simulink model "inerter_NL2"  (R2024b)
settings: Solver=ode1be  StartTime=0.0  StopTime=20  FixedStep=0.001  MaxStep=1e-2  MinStep=1e-12  RelTol=1e-6  AbsTol=1e-6
libraries: fl_lib x19, nesl_utility x7, simulink x1
settings Model: Creator=yl14470  LastModifiedBy=vzlat
settings SolverCC: MaxConsecutiveZCs=10000  ZeroCrossAlgorithm=Adaptive
settings DebuggingCC: IgnoredZcDiagnostic=none
settings RTWCC: GPUComputeCapability=3.5

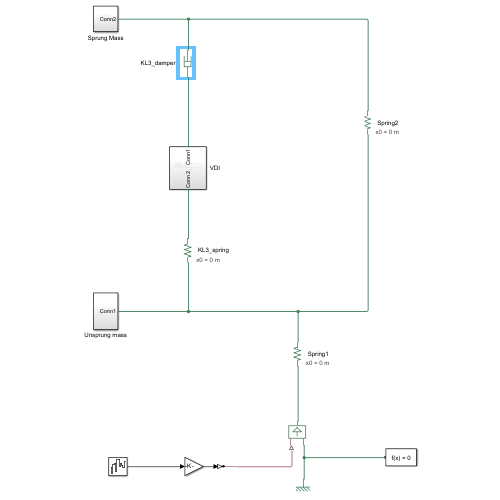
[thumbnail: Simulink's stored preview of the top-level diagram]
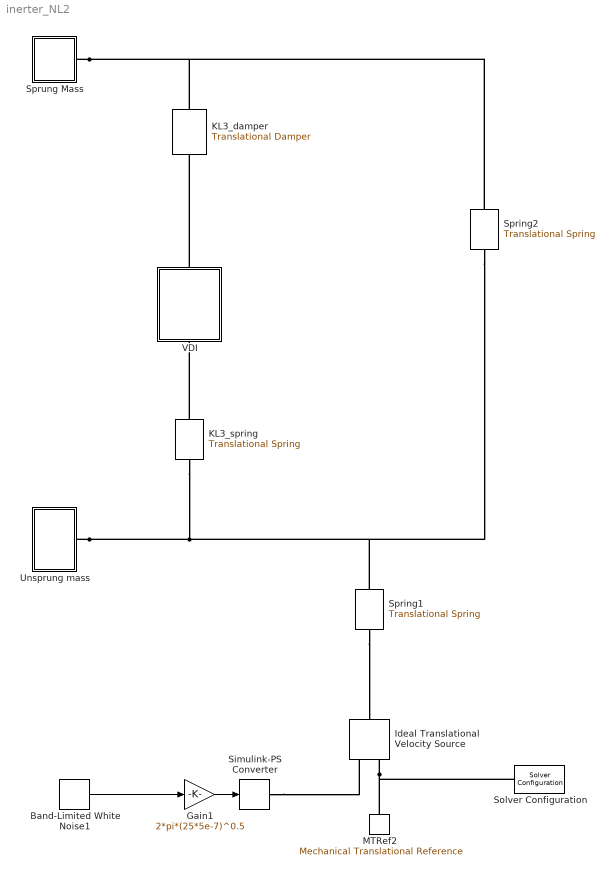
== system inerter_NL2 ==
  Band-Limited White Noise1 : simulink/Sources/Band-Limited White Noise  Cov=1  Ts=0.01  seed=[23341]
  Gain1 : Gain  Gain=2*pi*(25*5e-7)^0.5
  Ideal Translational Velocity Source : fl_lib/Mechanical/Mechanical Sources/Ideal Translational Velocity Source
  KL3_damper : fl_lib/Mechanical/Translational Elements/Translational Damper  D=962 N*s/m  v_specify=off  v_priority=None  v=0 m/s  v_nominal_specify=off  v_nominal_value=1  v_nominal_unit=m/s  f_specify=off  f_priority=None  f=0 N  f_nominal_specify=off  f_nominal_value=1  f_nominal_unit=N
  KL3_spring : fl_lib/Mechanical/Translational Elements/Translational Spring  spr_rate=10808 N/m  v_specify=off  v_priority=High  v=0 m/s  v_nominal_specify=off  v_nominal_value=1  v_nominal_unit=m/s  f_specify=off  f_priority=High  f=0 N  f_nominal_specify=off  f_nominal_value=1  f_nominal_unit=N  x_specify=on  x_priority=High  x=0 m  x_nominal_specify=off  x_nominal_value=1  x_nominal_unit=m
      settings: AttributesFormatString=x0 = %<x> %<x_unit>
  MTRef2 : fl_lib/Mechanical/Translational Elements/Mechanical Translational Reference
  Simulink-PS Converter : nesl_utility/Simulink-PS Converter  PhysicalDomain=network_engine_domain  SubClassName=ps_input  LeftPortType=input  RightPortType=output  PseudoPeriodic=off  Frequencies=[]  NoiseDistribution=none  NoiseParameters=[]  Unit=m/s  AffineConversion=off  FilteringAndDerivatives=filter  SimscapeFilterOrder=1  InputFilterTimeConstant=0.001  UdotUserProvided=0
  Solver Configuration : nesl_utility/Solver Configuration  PhysicalDomain=network_engine_domain  SubClassName=solver  LeftPortType=input  RightPortType=generic  Tones=[]  Harmonics=[]  SimulateNoise=off  Profile=off  UseLocalSampling=off  EnableSwitchedLinearOptims=on  FrequencyDomain=off  UseCCode=off  RelTol=0.001  AbsTol=1e-06  MinStep=1e-09  ToWorkspace=off  RevertToSquareIcSolve=off  NumHomotopyIterations=100  PhasorMode=off  PhasorModeNumHarmonics=1  ConsistencySolver=NEWTON_FTOL  IndexReductionMethod=DerivativeReplacement  DoDC=off  ResidualTolerance=1e-9  ConsistencyTolSource=GLOBAL  ConsistencyAbsTol=0.001  ConsistencyRelTol=0.001  ConsistencyTolFactor=0.001  UseLocalSolver=off  LocalSolverChoice=NE_BACKWARD_EULER_ADVANCER  ResolveIndetEquations=on  FunctionEvalNumThread=1  LocalSolverSampleTime=.001  DoFixedCost=off  MaxNonlinIter=12  MaxModeIter=2  ComputeImpulses=off  ImpulseIterations=2  LinearAlgebra=Sparse  LinearAlgebraNumThread=0  EquationFormulation=NE_TIME_EF  DelaysMemoryBudget=1024  AutomaticFiltering=on  FilteringTimeConstant=0.001  PartitionStorageMethod=AS_NEEDED  PartitionMemoryBudget=1024  PartitionMethod=FAST  MultibodyUseLocalSolver=off  MultibodyLocalSolverChoice=ODE1  MultibodyLocalSolverSampleTime=0.001
  Spring1 : fl_lib/Mechanical/Translational Elements/Translational Spring  spr_rate=160000 N/m  v_specify=off  v_priority=High  v=0 m/s  v_nominal_specify=off  v_nominal_value=1  v_nominal_unit=m/s  f_specify=off  f_priority=High  f=0 N  f_nominal_specify=off  f_nominal_value=1  f_nominal_unit=N  x_specify=on  x_priority=High  x=0 m  x_nominal_specify=off  x_nominal_value=1  x_nominal_unit=m
      settings: AttributesFormatString=x0 = %<x> %<x_unit>
  Spring2 : fl_lib/Mechanical/Translational Elements/Translational Spring  spr_rate=16998.2107 N/m  v_specify=off  v_priority=High  v=0 m/s  v_nominal_specify=off  v_nominal_value=1  v_nominal_unit=m/s  f_specify=off  f_priority=High  f=0 N  f_nominal_specify=off  f_nominal_value=1  f_nominal_unit=N  x_specify=on  x_priority=High  x=0 m  x_nominal_specify=off  x_nominal_value=1  x_nominal_unit=m
      settings: AttributesFormatString=x0 = %<x> %<x_unit>
  Sprung Mass : Subsystem
  Unsprung mass : Subsystem
  VDI : Subsystem
  wires:
  Gain1/1 -> Simulink-PS Converter/1
  Band-Limited White Noise1/1 -> Gain1/1
  connections:
  Sprung Mass/RConn1 -- Spring2/LConn1 -- KL3_damper/LConn1
  Unsprung mass/RConn1 -- Spring1/LConn1 -- Spring2/RConn1 -- KL3_spring/RConn1
  Ideal Translational Velocity Source/RConn2 -- MTRef2/LConn1 -- Solver Configuration/RConn1
  Spring1/RConn1 -- Ideal Translational Velocity Source/LConn1
  Simulink-PS Converter/RConn1 -- Ideal Translational Velocity Source/RConn1
  KL3_spring/LConn1 -- VDI/LConn1
  VDI/RConn1 -- KL3_damper/RConn1

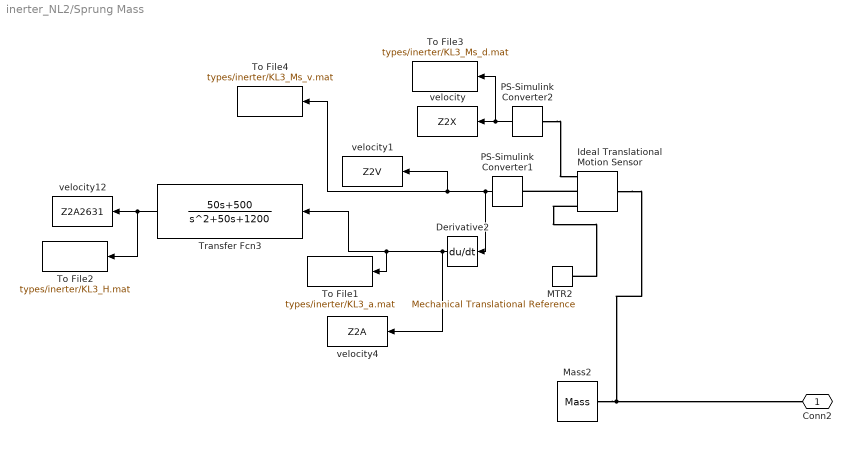
== system inerter_NL2/Sprung Mass ==
  Derivative2 : Derivative
  Ideal Translational Motion Sensor : fl_lib/Mechanical/Mechanical Sensors/Ideal Translational Motion Sensor  reference=foundation.enum.MeasurementReference.difference  acceleration_port=false  velocity_port=true  position_port=true  offset=0 m
  MTR2 : fl_lib/Mechanical/Translational Elements/Mechanical Translational Reference
  Mass2 : fl_lib/Mechanical/Translational Elements/Mass  mass=240 kg  num_ports=foundation.enum.numPorts2.one  v_specify=off  v_priority=High  v=0 m/s  v_nominal_specify=off  v_nominal_value=1  v_nominal_unit=m/s  f_specify=off  f_priority=High  f=0 N  f_nominal_specify=off  f_nominal_value=1  f_nominal_unit=N
  PS-Simulink Converter1 : nesl_utility/PS-Simulink Converter  PhysicalDomain=network_engine_domain  SubClassName=ps_output  LeftPortType=input  RightPortType=output  PseudoPeriodic=off  Frequencies=[]  VectorFormat=1-D array  Unit=1  AffineConversion=off
  PS-Simulink Converter2 : nesl_utility/PS-Simulink Converter  PhysicalDomain=network_engine_domain  SubClassName=ps_output  LeftPortType=input  RightPortType=output  PseudoPeriodic=off  Frequencies=[]  VectorFormat=1-D array  Unit=1  AffineConversion=off
  To File1 : ToFile  Filename=types/inerter/KL3_a.mat  MatrixName=Ms_acc  SaveFormat=Timeseries
  To File2 : ToFile  Filename=types/inerter/KL3_H.mat  MatrixName=H2631  SaveFormat=Timeseries
  To File3 : ToFile  Filename=types/inerter/KL3_Ms_d.mat  MatrixName=Ms_d  SaveFormat=Timeseries
  To File4 : ToFile  Filename=types/inerter/KL3_Ms_v.mat  MatrixName=Ms_v  SaveFormat=Timeseries
  Transfer Fcn3 : TransferFcn  Numerator=[0 50 500]  Denominator=[1 50 1200]
  velocity : ToWorkspace  VariableName=Z2X  SampleTime=-1
  velocity1 : ToWorkspace  VariableName=Z2V  SampleTime=-1
  velocity12 : ToWorkspace  VariableName=Z2A2631  SampleTime=-1
  velocity4 : ToWorkspace  VariableName=Z2A  SampleTime=-1
  Conn2 : PMIOPort  Side=Right
  wires:
  Transfer Fcn3/1 -> To File2/1, velocity12/1
  PS-Simulink Converter1/1 -> Derivative2/1, To File4/1, velocity1/1
  Derivative2/1 -> To File1/1, Transfer Fcn3/1, velocity4/1
  PS-Simulink Converter2/1 -> velocity/1, To File3/1
  connections:
  Ideal Translational Motion Sensor/RConn1 -- MTR2/LConn1
  Mass2/LConn1 -- Conn2/RConn1 -- Ideal Translational Motion Sensor/LConn1
  Ideal Translational Motion Sensor/RConn2 -- PS-Simulink Converter1/LConn1
  PS-Simulink Converter2/LConn1 -- Ideal Translational Motion Sensor/RConn3

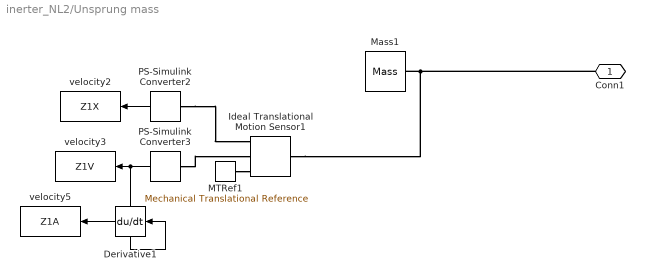
== system inerter_NL2/Unsprung mass ==
  Derivative1 : Derivative
  Ideal Translational Motion Sensor1 : fl_lib/Mechanical/Mechanical Sensors/Ideal Translational Motion Sensor  reference=foundation.enum.MeasurementReference.difference  acceleration_port=false  velocity_port=true  position_port=true  offset=0 m
  MTRef1 : fl_lib/Mechanical/Translational Elements/Mechanical Translational Reference
  Mass1 : fl_lib/Mechanical/Translational Elements/Mass  mass=36 kg  num_ports=foundation.enum.numPorts2.one  v_specify=off  v_priority=High  v=0 m/s  v_nominal_specify=off  v_nominal_value=1  v_nominal_unit=m/s  f_specify=off  f_priority=High  f=0 N  f_nominal_specify=off  f_nominal_value=1  f_nominal_unit=N
  PS-Simulink Converter2 : nesl_utility/PS-Simulink Converter  PhysicalDomain=network_engine_domain  SubClassName=ps_output  LeftPortType=input  RightPortType=output  PseudoPeriodic=off  Frequencies=[]  VectorFormat=1-D array  Unit=1  AffineConversion=off
  PS-Simulink Converter3 : nesl_utility/PS-Simulink Converter  PhysicalDomain=network_engine_domain  SubClassName=ps_output  LeftPortType=input  RightPortType=output  PseudoPeriodic=off  Frequencies=[]  VectorFormat=1-D array  Unit=1  AffineConversion=off
  velocity2 : ToWorkspace  VariableName=Z1X  SampleTime=-1
  velocity3 : ToWorkspace  VariableName=Z1V  SampleTime=-1
  velocity5 : ToWorkspace  VariableName=Z1A  SampleTime=-1
  Conn1 : PMIOPort  Side=Right
  wires:
  PS-Simulink Converter3/1 -> velocity3/1, Derivative1/1
  Derivative1/1 -> velocity5/1
  PS-Simulink Converter2/1 -> velocity2/1
  connections:
  Mass1/LConn1 -- Conn1/RConn1 -- Ideal Translational Motion Sensor1/LConn1
  MTRef1/LConn1 -- Ideal Translational Motion Sensor1/RConn1
  PS-Simulink Converter3/LConn1 -- Ideal Translational Motion Sensor1/RConn2
  PS-Simulink Converter2/LConn1 -- Ideal Translational Motion Sensor1/RConn3

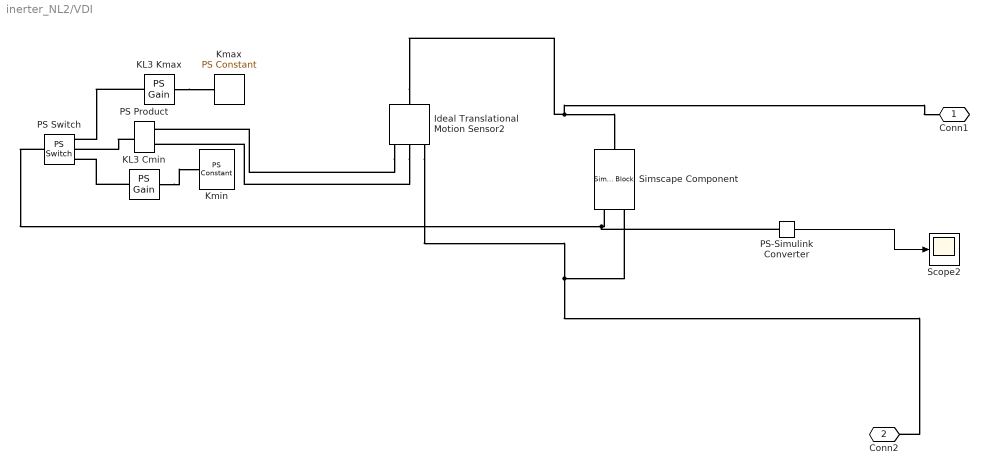
== system inerter_NL2/VDI ==
  Ideal Translational Motion Sensor2 : fl_lib/Mechanical/Mechanical Sensors/Ideal Translational Motion Sensor  reference=foundation.enum.MeasurementReference.difference  acceleration_port=false  velocity_port=true  position_port=true  offset=0 m
  KL3 Cmin : fl_lib/Physical Signals/Functions/PS Gain  gain=1
  KL3 Kmax : fl_lib/Physical Signals/Functions/PS Gain  gain=1
  Kmax : fl_lib/Physical Signals/Sources/PS Constant  constant=177 kg
  Kmin : fl_lib/Physical Signals/Sources/PS Constant  constant=68 kg
  PS Product : fl_lib/Physical Signals/Functions/PS Product
  PS Switch : fl_lib/Physical Signals/Nonlinear Operators/PS Switch  Threshold=0 m^2/s
      settings: InternalSimscapePortConfiguration="{\"Bottom\":[],\"Left\":[{\"id\":\"I1\",\"label\":\"\",\"type\":\"input\"},{\"id\":\"I2\",\"label\":\"\",\"type\":\"input\"},{\"id\":\"I3\",\"label\":\"\",\"type\":\"input\"}],\"Right\":[{\"id\":\"O\",\"label\":\"\",\"type\":\"output\"}],\"Top\":[]}"
  PS-Simulink Converter : nesl_utility/PS-Simulink Converter  PhysicalDomain=network_engine_domain  SubClassName=ps_output  LeftPortType=input  RightPortType=output  PseudoPeriodic=off  Frequencies=[]  VectorFormat=inherit  Unit=inherit  AffineConversion=off
  Scope2 : Scope
  Simscape Component : SimscapeComponentBlock  SourceFile=component_with_input  ComponentPath=component_with_input  ComponentVariants="[\"component_with_input\"]"  ComponentVariantNames="[\"component_with_input\"]"  ClassName=component_with_input  SchemaVersion=1  Bmin=1 kg  v_specify=off  v_priority=High  v=0 m/s  v_nominal_specify=off  v_nominal_value=1  v_nominal_unit=m/s  f_specify=off  f_priority=None  f=0 N  f_nominal_specify=off  f_nominal_value=1  f_nominal_unit=N
      settings: CopyFcn=simscape.engine.sli.internal.componentblockcallback(gcbh,'COPY')  PreCopyFcn=simscape.engine.sli.internal.componentblockcallback(gcbh,'PRECOPY')  PreDeleteFcn=simscape.engine.sli.internal.componentblockcallback(gcbh,'PREDELETE')  InternalSimscapePortConfiguration="{\"Bottom\":[],\"Left\":[{\"id\":\"B\",\"label\":\"K\",\"type\":\"input\"},{\"id\":\"R\",\"label\":\"R\",\"type\":\"foundation.mechanical.translational.translational\"}],\"Right\":[{\"id\":\"C\",\"label\":\"C\",\"type\":\"foundation.mechanical.translational.translational\"}],\"Top\":[]}"
      mask Type: Translational Inerter
  Conn1 : PMIOPort  Side=Right
  Conn2 : PMIOPort  Port=2  Side=Left
  wires:
  PS-Simulink Converter/1 -> Scope2/1
  connections:
  Ideal Translational Motion Sensor2/RConn3 -- PS Product/LConn2
  Ideal Translational Motion Sensor2/RConn1 -- Simscape Component/LConn2 -- Conn2/RConn1
  Ideal Translational Motion Sensor2/LConn1 -- Simscape Component/RConn1 -- Conn1/RConn1
  KL3 Cmin/LConn1 -- Kmin/RConn1
  PS Product/RConn1 -- PS Switch/LConn2
  KL3 Cmin/RConn1 -- PS Switch/LConn1
  KL3 Kmax/RConn1 -- PS Switch/LConn3
  KL3 Kmax/LConn1 -- Kmax/RConn1
  Ideal Translational Motion Sensor2/RConn2 -- PS Product/LConn1
  PS Switch/RConn1 -- PS-Simulink Converter/LConn1 -- Simscape Component/LConn1
